simulink model "Kinematic_Consensus"  (R2025a)
settings: Solver=VariableStepAuto  StartTime=0.0  StopTime=50  RelTol=1e-3
settings Model: Creator=huy01  LastModifiedBy=huy01

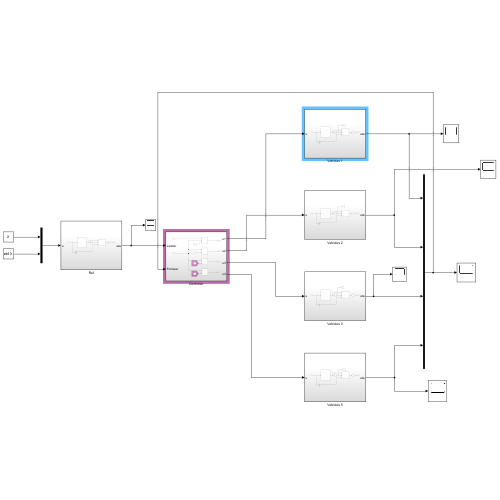
[thumbnail: Simulink's stored preview of the top-level diagram]
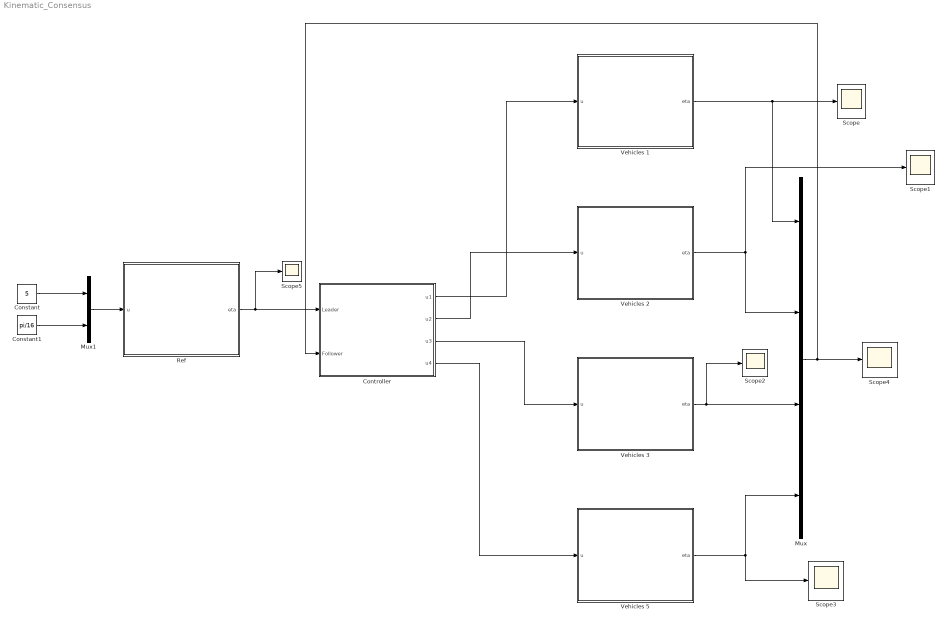
== system Kinematic_Consensus ==
  Constant : Constant  Value=5
  Constant1 : Constant  Value=pi/16
  Controller : Subsystem
  Mux : Mux
  Mux1 : Mux  Inputs=2
  Ref : Subsystem
  Scope{,1..5} (6 alike) : Scope
      Scope settings: ActiveDisplayYMinimum=-38.91222933725517  ActiveDisplayYMaximum=44.45409734017278
      Scope2 settings: DataLoggingVariableName=ScopeData2
      Scope3 settings: ActiveDisplayYMinimum=-172.42763448595133  ActiveDisplayYMaximum=108.05419123294409  DataLoggingVariableName=ScopeData3
      Scope4 settings: ActiveDisplayYMinimum=-95.71421877007802  ActiveDisplayYMaximum=91.130505863862879  DataLoggingVariableName=ScopeData4
      Scope5 settings: ActiveDisplayYMinimum=-1  ActiveDisplayYMaximum=1  DataLoggingVariableName=ScopeData5
  Vehicles 1 : Subsystem
  Vehicles 2 : Subsystem
  Vehicles 3 : Subsystem
  Vehicles 5 : Subsystem
  wires:
  Vehicles 5/1(eta) -> Scope3/1, Mux/4
  Vehicles 3/1(eta) -> Mux/3, Scope2/1
  Vehicles 1/1(eta) -> Scope/1, Mux/1
  Mux/1 -> Scope4/1, Controller/2(Follower)
  Ref/1(eta) -> Scope5/1, Controller/1(Leader)
  Vehicles 2/1(eta) -> Scope1/1, Mux/2
  Controller/1(u1) -> Vehicles 1/1(u)
  Controller/2(u2) -> Vehicles 2/1(u)
  Controller/3(u3) -> Vehicles 3/1(u)
  Controller/4(u4) -> Vehicles 5/1(u)
  Mux1/1 -> Ref/1(u)
  Constant/1 -> Mux1/1
  Constant1/1 -> Mux1/2

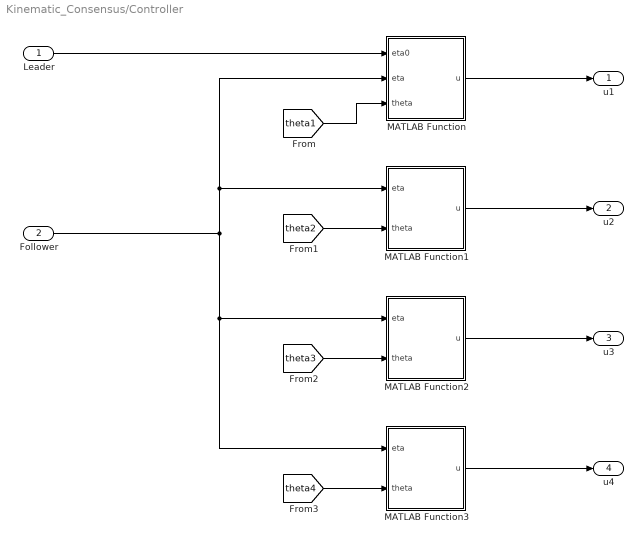
== system Kinematic_Consensus/Controller ==
  Leader : Inport
  Follower : Inport  Port=2
  MATLAB Function : MATLAB Function  TreatAsAtomicUnit=on
  MATLAB Function1 : MATLAB Function  TreatAsAtomicUnit=on
  MATLAB Function2 : MATLAB Function  TreatAsAtomicUnit=on
  MATLAB Function3 : MATLAB Function  TreatAsAtomicUnit=on
  u1 : Outport
  u2 : Outport  Port=2
  u3 : Outport  Port=3
  u4 : Outport  Port=4
  wires:
  MATLAB Function/1(u) -> u1/1
  Leader/1 -> MATLAB Function/1(eta0)
  Follower/1 -> MATLAB Function2/1(eta), MATLAB Function3/1(eta), MATLAB Function1/1(eta), MATLAB Function/2(eta)
  MATLAB Function1/1(u) -> u2/1
  MATLAB Function2/1(u) -> u3/1
  MATLAB Function3/1(u) -> u4/1
  [theta1] -> MATLAB Function/3(theta)
  [theta2] -> MATLAB Function1/2(theta)
  [theta3] -> MATLAB Function2/2(theta)
  [theta4] -> MATLAB Function3/2(theta)

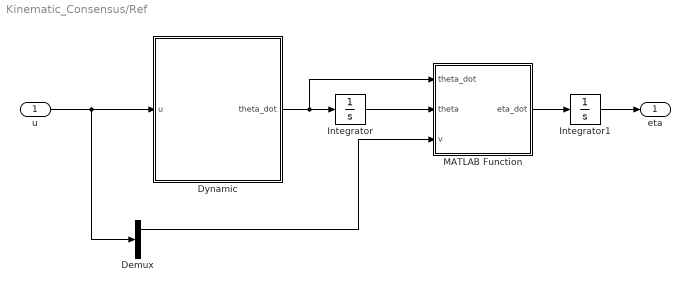
== system Kinematic_Consensus/Ref ==
  u : Inport
  Demux : Demux  Outputs=2
  Dynamic : MATLAB Function  TreatAsAtomicUnit=on
  Integrator : Integrator  InitialCondition=2*pi/3
  Integrator1 : Integrator  InitialCondition=[35;-5]
  MATLAB Function : MATLAB Function  TreatAsAtomicUnit=on
  eta : Outport
  wires:
  u/1 -> Demux/1, Dynamic/1(u)
  Dynamic/1(theta_dot) -> MATLAB Function/1(theta_dot), Integrator/1
  Integrator/1 -> MATLAB Function/2(theta)
  MATLAB Function/1(eta_dot) -> Integrator1/1
  Integrator1/1 -> eta/1
  Demux/1 -> MATLAB Function/3(v)

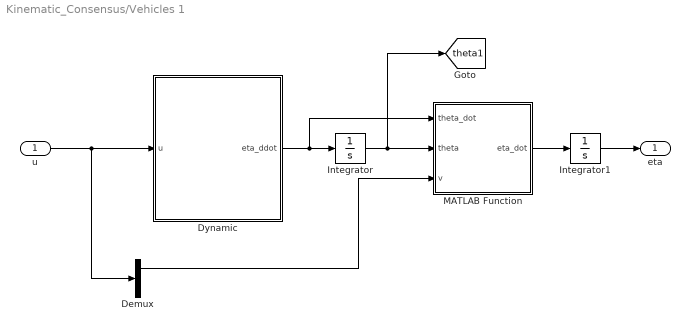
== system Kinematic_Consensus/Vehicles 1 ==
  u : Inport
  Demux : Demux  Outputs=2
  Dynamic : MATLAB Function  TreatAsAtomicUnit=on
  Integrator : Integrator  InitialCondition=pi/2
  Integrator1 : Integrator  InitialCondition=[25;5]
  MATLAB Function : MATLAB Function  TreatAsAtomicUnit=on
  eta : Outport
  tag scope: theta1=global
  wires:
  u/1 -> Demux/1, Dynamic/1(u)
  Dynamic/1(eta_ddot) -> MATLAB Function/1(theta_dot), Integrator/1
  Integrator/1 -> [theta1], MATLAB Function/2(theta)
  MATLAB Function/1(eta_dot) -> Integrator1/1
  Integrator1/1 -> eta/1
  Demux/1 -> MATLAB Function/3(v)

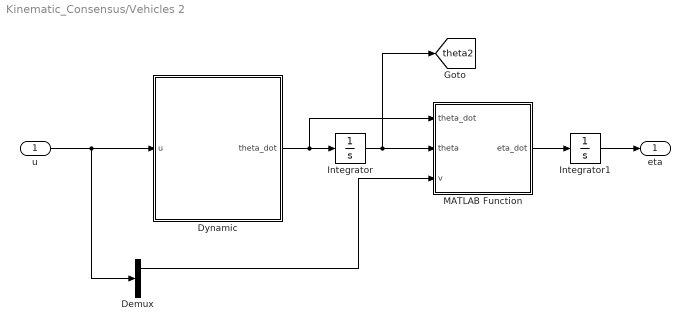
== system Kinematic_Consensus/Vehicles 2 ==
  u : Inport
  Demux : Demux  Outputs=2
  Dynamic : MATLAB Function  TreatAsAtomicUnit=on
  Integrator : Integrator
  Integrator1 : Integrator  InitialCondition=[20;10]
  MATLAB Function : MATLAB Function  TreatAsAtomicUnit=on
  eta : Outport
  tag scope: theta2=global
  wires:
  u/1 -> Demux/1, Dynamic/1(u)
  Dynamic/1(theta_dot) -> MATLAB Function/1(theta_dot), Integrator/1
  Integrator/1 -> [theta2], MATLAB Function/2(theta)
  MATLAB Function/1(eta_dot) -> Integrator1/1
  Integrator1/1 -> eta/1
  Demux/1 -> MATLAB Function/3(v)

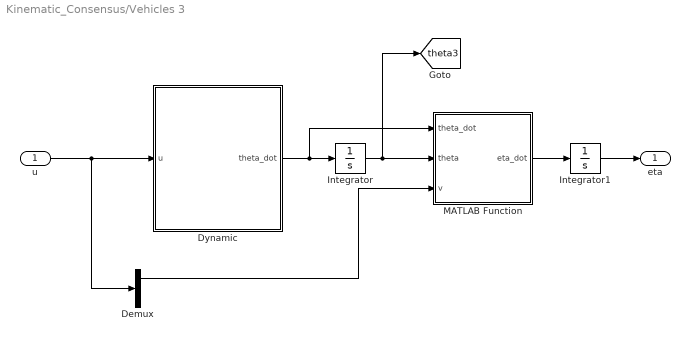
== system Kinematic_Consensus/Vehicles 3 ==
  u : Inport
  Demux : Demux  Outputs=2
  Dynamic : MATLAB Function  TreatAsAtomicUnit=on
  Integrator : Integrator
  Integrator1 : Integrator  InitialCondition=[10;10]
  MATLAB Function : MATLAB Function  TreatAsAtomicUnit=on
  eta : Outport
  tag scope: theta3=global
  wires:
  u/1 -> Demux/1, Dynamic/1(u)
  Dynamic/1(theta_dot) -> MATLAB Function/1(theta_dot), Integrator/1
  Integrator/1 -> [theta3], MATLAB Function/2(theta)
  MATLAB Function/1(eta_dot) -> Integrator1/1
  Integrator1/1 -> eta/1
  Demux/1 -> MATLAB Function/3(v)

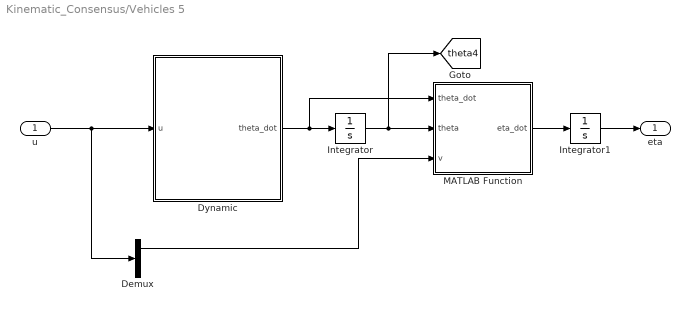
== system Kinematic_Consensus/Vehicles 5 ==
  u : Inport
  Demux : Demux  Outputs=2
  Dynamic : MATLAB Function  TreatAsAtomicUnit=on
  Integrator : Integrator  InitialCondition=pi/3
  Integrator1 : Integrator  InitialCondition=[5;5]
  MATLAB Function : MATLAB Function  TreatAsAtomicUnit=on
  eta : Outport
  tag scope: theta4=global
  wires:
  u/1 -> Demux/1, Dynamic/1(u)
  Dynamic/1(theta_dot) -> MATLAB Function/1(theta_dot), Integrator/1
  Integrator/1 -> [theta4], MATLAB Function/2(theta)
  MATLAB Function/1(eta_dot) -> Integrator1/1
  Integrator1/1 -> eta/1
  Demux/1 -> MATLAB Function/3(v)

== matlab function Kinematic_Consensus/Controller/MATLAB Function2 ==
  data: u output; eta input; theta input
function u = fcn(eta, theta)
    r = 5;
    muy = 1.7;
    
    u1 = -muy*(2.*[eta(5); eta(6)] - [eta(3); eta(4)] - [eta(7); eta(8)]);

    v = u1(1)*cos(theta) + u1(2)*sin(theta);
    phi = atan((-u1(1)*sin(theta)/r + u1(2)*cos(theta)/r)/u1(1));

    u = [v; phi];

end

== matlab function Kinematic_Consensus/Controller/MATLAB Function3 ==
  data: u output; eta input; theta input
function u = fcn(eta, theta)
    r = 5;
    muy = 1.7;

    u1 = -muy*(2.*[eta(7); eta(8)] - [eta(3); eta(4)] - [eta(5); eta(6)]);

    v = u1(1)*cos(theta) + u1(2)*sin(theta);
    phi = atan((-u1(1)*sin(theta)/r + u1(2)*cos(theta)/r)/u1(1));

    u = [v; phi];

end

== matlab function Kinematic_Consensus/Vehicles 1/Dynamic ==
  data: u input size=[2;1]; eta_ddot output
function eta_ddot = fcn(u)

    eta_ddot = u;

end

== matlab function Kinematic_Consensus/Vehicles 2/Dynamic ==
  data: u input; theta_dot output
function theta_dot = fcn(u)

    theta_dot = u(1)*tan(u(2));

end

== matlab function Kinematic_Consensus/Vehicles 2/MATLAB Function ==
  data: theta_dot input; theta input; eta_dot output; v input
function eta_dot = fcn(theta_dot, theta, v)

    r = 5;

    xC_dot = v*cos(theta) - theta_dot*r*sin(theta);
    yC_dot = v*sin(theta) + theta_dot*r*cos(theta);

    eta_dot = [xC_dot; yC_dot];

end

== matlab function Kinematic_Consensus/Vehicles 3/Dynamic ==
  data: u input; theta_dot output
function theta_dot = fcn(u)

    theta_dot = u(1)*tan(u(2));

end

== matlab function Kinematic_Consensus/Vehicles 3/MATLAB Function ==
  data: theta_dot input; theta input; eta_dot output; v input
function eta_dot = fcn(theta_dot, theta, v)

    r = 5;

    xC_dot = v*cos(theta) - theta_dot*r*sin(theta);
    yC_dot = v*sin(theta) + theta_dot*r*cos(theta);

    eta_dot = [xC_dot; yC_dot];

end

== matlab function Kinematic_Consensus/Controller/MATLAB Function ==
  data: eta0 input; u output; eta input; theta input
function u = fcn(eta0, eta, theta)
    r = 5;
    muy = 1.7;

    u1 = -muy*([eta(1); eta(2)] - [eta(3); eta(4)]) - muy*([eta(1); eta(2)] - [eta0(1); eta0(2)]);

    v = u1(1)*cos(theta) + u1(2)*sin(theta);
    phi = atan((-u1(1)*sin(theta)/r + u1(2)*cos(theta)/r)/u1(1));

    u = [v; phi];

end

== matlab function Kinematic_Consensus/Ref/Dynamic ==
  data: u input; theta_dot output
function theta_dot = fcn(u)

    theta_dot = u(1)*tan(u(2));

end

== matlab function Kinematic_Consensus/Ref/MATLAB Function ==
  data: theta_dot input; theta input; eta_dot output; v input
function eta_dot = fcn(theta_dot, theta, v)

    r = 5;

    xC_dot = v*cos(theta) - theta_dot*r*sin(theta);
    yC_dot = v*sin(theta) + theta_dot*r*cos(theta);

    eta_dot = [xC_dot; yC_dot];

end

== matlab function Kinematic_Consensus/Vehicles 5/Dynamic ==
  data: u input; theta_dot output
function theta_dot = fcn(u)

    theta_dot = u(1)*tan(u(2));

end

== matlab function Kinematic_Consensus/Vehicles 5/MATLAB Function ==
  data: theta_dot input; theta input; eta_dot output; v input
function eta_dot = fcn(theta_dot, theta, v)

    r = 5;

    xC_dot = v*cos(theta) - theta_dot*r*sin(theta);
    yC_dot = v*sin(theta) + theta_dot*r*cos(theta);

    eta_dot = [xC_dot; yC_dot];

end

== matlab function Kinematic_Consensus/Vehicles 1/MATLAB Function ==
  data: theta_dot input; theta input; eta_dot output; v input
function eta_dot = fcn(theta_dot, theta, v)

    r = 5;

    xC_dot = v*cos(theta) - theta_dot*r*sin(theta);
    yC_dot = v*sin(theta) + theta_dot*r*cos(theta);

    eta_dot = [xC_dot; yC_dot];

end

== matlab function Kinematic_Consensus/Controller/MATLAB Function1 ==
  data: u output; eta input; theta input
function u = fcn(eta, theta)
    r = 5;
    muy = 1.7;

    u1 = -muy*(3.*[eta(3); eta(4)] - [eta(1); eta(2)] - [eta(5); eta(6)] - [eta(7); eta(8)]);

    v = u1(1)*cos(theta) + u1(2)*sin(theta);
    phi = atan((-u1(1)*sin(theta)/r + u1(2)*cos(theta)/r)/u1(1));

    u = [v; phi];

end
